simulink model "PIDmodelosimples"  (R2023a)
settings: Solver=FixedStepAuto  StartTime=0.0  StopTime=3  FixedStep=1e-5  RelTol=1e-3
settings Model: Creator=a2150336  LastModifiedBy=a2150336

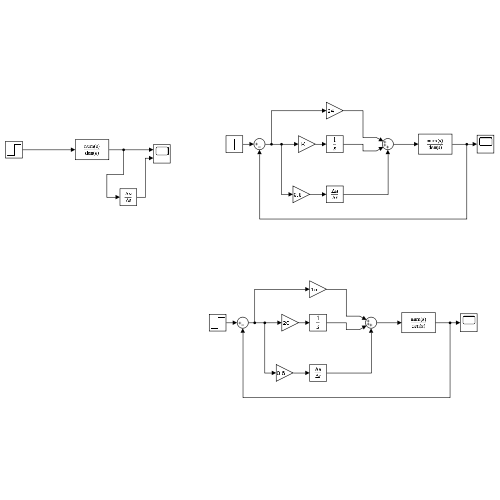
[thumbnail: Simulink's stored preview of the top-level diagram]
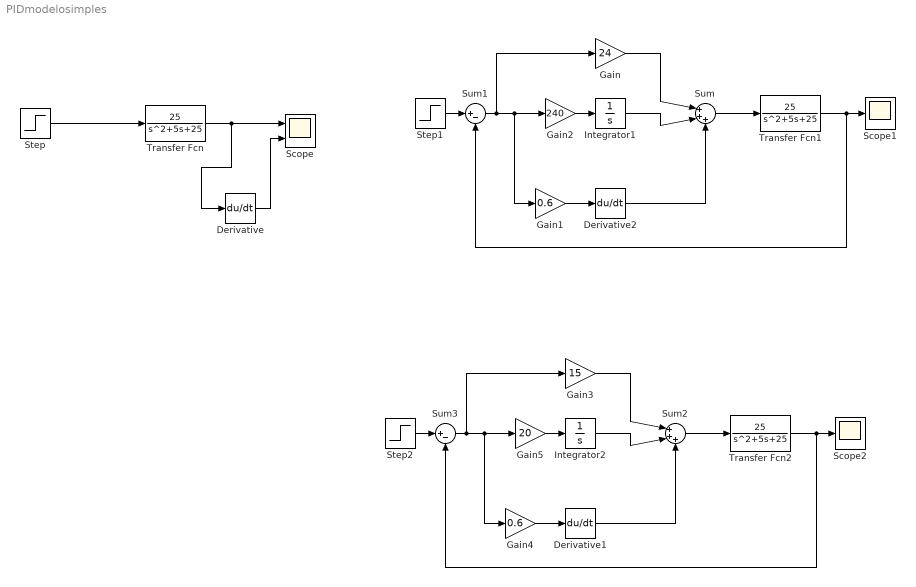
== system PIDmodelosimples ==
  Derivative : Derivative
  Derivative1 : Derivative
  Derivative2 : Derivative
  Gain : Gain  Gain=24
  Gain1 : Gain  Gain=0.6
  Gain2 : Gain  Gain=240
  Gain3 : Gain  Gain=15
  Gain4 : Gain  Gain=0.6
  Gain5 : Gain  Gain=20
  Integrator1 : Integrator
  Integrator2 : Integrator
  Scope : Scope  NumInputPorts=2
  Scope1 : Scope
  Scope2 : Scope
  Step : Step  SampleTime=0
  Step1 : Step  SampleTime=0
  Step2 : Step  SampleTime=0
  Sum : Sum  Inputs=|+++
  Sum1 : Sum  Inputs=|+-
  Sum2 : Sum  Inputs=|+++
  Sum3 : Sum  Inputs=|+-
  Transfer Fcn : TransferFcn  Numerator=[25]  Denominator=[1 5 25]
  Transfer Fcn1 : TransferFcn  Numerator=[25]  Denominator=[1 5 25]
  Transfer Fcn2 : TransferFcn  Numerator=[25]  Denominator=[1 5 25]
  wires:
  Transfer Fcn/1 -> Derivative/1, Scope/1
  Step/1 -> Transfer Fcn/1
  Derivative/1 -> Scope/2
  Transfer Fcn1/1 -> Scope1/1, Sum1/2
  Sum/1 -> Transfer Fcn1/1
  Gain2/1 -> Integrator1/1
  Gain1/1 -> Derivative2/1
  Gain/1 -> Sum/1
  Integrator1/1 -> Sum/2
  Derivative2/1 -> Sum/3
  Step1/1 -> Sum1/1
  Sum1/1 -> Gain/1, Gain1/1, Gain2/1
  Gain3/1 -> Sum2/1
  Sum2/1 -> Transfer Fcn2/1
  Gain4/1 -> Derivative1/1
  Derivative1/1 -> Sum2/3
  Gain5/1 -> Integrator2/1
  Sum3/1 -> Gain3/1, Gain4/1, Gain5/1
  Transfer Fcn2/1 -> Scope2/1, Sum3/2
  Integrator2/1 -> Sum2/2
  Step2/1 -> Sum3/1
